simulink model "motor_simu"  (Simulink 7.7)
settings: Solver=ode45  StartTime=0.0  StopTime=100
values from neighbouring files (symbols this model uses):
  b = Cubesatmotorb    [main.m]
  J = Cubesatmotorrotorinertia    [main.m]
  Jc = structureinertiaJzz    [main.m]
  Jri = ((Cubesatmotorrotorinertia) + (flywheelinertiaJzz))    [main.m]
  Ke = CubesatmotorSconst    [main.m]
  Kt = CubesatmotorTconst    [main.m]
  L = CubesatmotorLrup    [main.m]
  R = CubesatmotorRrup    [main.m]
libraries: simulink x2
settings Model: Creator=Felipe  LastModifiedBy=user

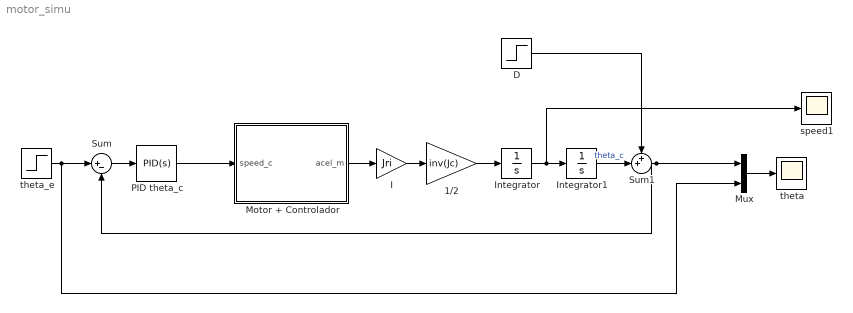
== system motor_simu ==
  1/2 : Gain  Gain=inv(Jc)
  D : Step  Time=150  After=(pi/4)/10  SampleTime=0
  I : Gain  Gain=Jri
  Integrator : Integrator
  Integrator1 : Integrator
  Motor + Controlador : Subsystem
  Mux : Mux  Inputs=2
  PID theta_c : simulink/Continuous/PID Controller  SystemSampleTime=-1  Controller=PID  TimeDomain=Continuous-time  SampleTime=1  IntegratorMethod=Forward Euler  FilterMethod=Forward Euler  Form=Parallel  P=4.2713440821133  I=0.2  D=-0.0891061021532855  N=47.9354834168987  InitialConditionSource=internal  InitialConditionForIntegrator=0  InitialConditionForFilter=0  ExternalReset=none  LimitOutput=off  UpperSaturationLimit=inf  LowerSaturationLimit=-inf  LinearizeAsGain=off  AntiWindupMode=none  Kb=1  TrackingMode=off  Kt=1  PParamMin=[]  PParamMax=[]  IParamMin=[]  IParamMax=[]  DParamMin=[]  DParamMax=[]  NParamMin=[]  NParamMax=[]  KbParamMin=[]  KbParamMax=[]  KtParamMin=[]  KtParamMax=[]  POutMin=[]  POutMax=[]  IOutMin=[]  IOutMax=[]  DOutMin=[]  DOutMax=[]  NOutMin=[]  NOutMax=[]  KbOutMin=[]  KbOutMax=[]  KtOutMin=[]  KtOutMax=[]  IntegratorOutMin=[]  IntegratorOutMax=[]  FilterOutMin=[]  FilterOutMax=[]  SumOutMin=[]  SumOutMax=[]  SumI1OutMin=[]  SumI1OutMax=[]  SumI2OutMin=[]  SumI2OutMax=[]  SumI3OutMin=[]  SumI3OutMax=[]  SumDOutMin=[]  SumDOutMax=[]  SaturationOutMin=[]  SaturationOutMax=[]  IntegratorContinuousStateAttributes=''  IntegratorStateMustResolveToSignalObject=off  IntegratorRTWStateStorageClass=Auto  FilterContinuousStateAttributes=''  FilterStateMustResolveToSignalObject=off  FilterRTWStateStorageClass=Auto
  Sum : Sum  Inputs=|+-
  Sum1 : Sum  Inputs=++|
  speed1 : Scope
      settings: SaveName=ScopeData3
  theta : Scope
      settings: YMin=-0.05  YMax=0.8
  theta_e : Step  After=(pi/4)  SampleTime=0
  wires:
  Motor + Controlador/1(acel_m) -> I/1
  I/1 -> 1/2/1
  Integrator/1 -> Integrator1/1, speed1/1
  PID theta_c/1 -> Motor + Controlador/1(speed_c)
  theta_e/1 -> Sum/1, Mux/2
  Sum/1 -> PID theta_c/1
  Mux/1 -> theta/1
  1/2/1 -> Integrator/1
  Integrator1/1 -> Sum1/2  "theta_c"
  D/1 -> Sum1/1
  Sum1/1 -> Sum/2, Mux/1

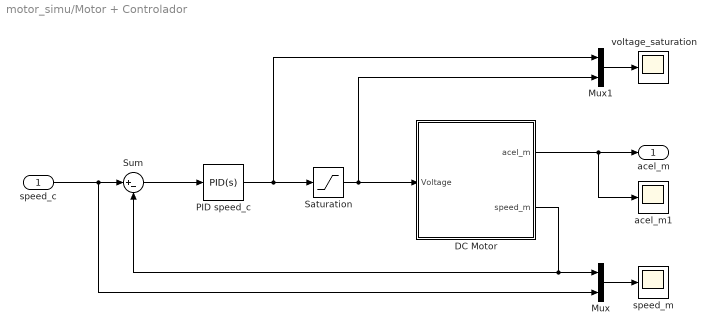
== system motor_simu/Motor + Controlador ==
  speed_c : Inport
  DC Motor : Subsystem
  Mux : Mux  Inputs=2
  Mux1 : Mux  Inputs=2
  PID speed_c : simulink/Continuous/PID Controller  SystemSampleTime=-1  Controller=PID  TimeDomain=Continuous-time  SampleTime=1  IntegratorMethod=Forward Euler  FilterMethod=Forward Euler  Form=Parallel  P=4.72772772635323  I=0.0083033953310603  D=-0.206120281132516  N=22.936742082715  InitialConditionSource=internal  InitialConditionForIntegrator=0  InitialConditionForFilter=0  ExternalReset=none  LimitOutput=off  UpperSaturationLimit=inf  LowerSaturationLimit=-inf  LinearizeAsGain=off  AntiWindupMode=none  Kb=1  TrackingMode=off  Kt=1  PParamMin=[]  PParamMax=[]  IParamMin=[]  IParamMax=[]  DParamMin=[]  DParamMax=[]  NParamMin=[]  NParamMax=[]  KbParamMin=[]  KbParamMax=[]  KtParamMin=[]  KtParamMax=[]  POutMin=[]  POutMax=[]  IOutMin=[]  IOutMax=[]  DOutMin=[]  DOutMax=[]  NOutMin=[]  NOutMax=[]  KbOutMin=[]  KbOutMax=[]  KtOutMin=[]  KtOutMax=[]  IntegratorOutMin=[]  IntegratorOutMax=[]  FilterOutMin=[]  FilterOutMax=[]  SumOutMin=[]  SumOutMax=[]  SumI1OutMin=[]  SumI1OutMax=[]  SumI2OutMin=[]  SumI2OutMax=[]  SumI3OutMin=[]  SumI3OutMax=[]  SumDOutMin=[]  SumDOutMax=[]  SaturationOutMin=[]  SaturationOutMax=[]  IntegratorContinuousStateAttributes=''  IntegratorStateMustResolveToSignalObject=off  IntegratorRTWStateStorageClass=Auto  FilterContinuousStateAttributes=''  FilterStateMustResolveToSignalObject=off  FilterRTWStateStorageClass=Auto
  Saturation : Saturate  UpperLimit=12  LowerLimit=-12
  Sum : Sum  Inputs=|+-
  acel_m1 : Scope
      settings: YMin=-0.095  YMax=0
  speed_m : Scope
      settings: SaveName=ScopeData2
  voltage_saturation : Scope
      settings: SaveName=ScopeData5
  acel_m : Outport
  wires:
  DC Motor/2(speed_m) -> Sum/2, Mux/1
  Saturation/1 -> DC Motor/1(Voltage), Mux1/2
  PID speed_c/1 -> Saturation/1, Mux1/1
  Sum/1 -> PID speed_c/1
  speed_c/1 -> Sum/1, Mux/2
  DC Motor/1(acel_m) -> acel_m/1, acel_m1/1
  Mux/1 -> speed_m/1
  Mux1/1 -> voltage_saturation/1

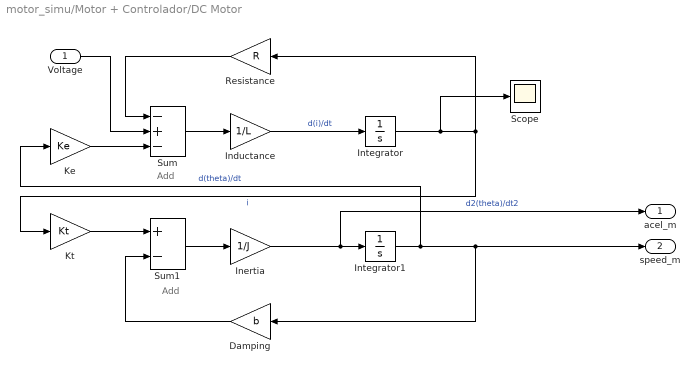
== system motor_simu/Motor + Controlador/DC Motor ==
  note: Add
  note: Add
  Voltage : Inport
  Damping : Gain  RequirementInfo={} %GIDa_a0bca8fb_deb2_4cd3_97cf_4f937a3969db  Gain=b
  Inductance : Gain  Gain=1/L
  Inertia : Gain  Gain=1/J
  Integrator : Integrator
  Integrator1 : Integrator
  Ke : Gain  Gain=Ke
  Kt : Gain  Gain=Kt
  Resistance : Gain  RequirementInfo={} %GIDa_06d63a89_88ab_48b6_b71f_14b802dc9c0a  Gain=R
  Scope : Scope
      settings: SaveName=ScopeData4
  Sum : Sum  Inputs=-+-
  Sum1 : Sum  Inputs=+-
  acel_m : Outport
  speed_m : Outport  Port=2
  wires:
  Resistance/1 -> Sum/1
  Voltage/1 -> Sum/2
  Ke/1 -> Sum/3
  Damping/1 -> Sum1/2
  Kt/1 -> Sum1/1
  Sum1/1 -> Inertia/1
  Sum/1 -> Inductance/1
  Inertia/1 -> Integrator1/1, acel_m/1  "d2(theta)/dt2"
  Integrator1/1 -> speed_m/1, Damping/1, Ke/1  "d(theta)/dt"
  Inductance/1 -> Integrator/1  "d(i)/dt"
  Integrator/1 -> Resistance/1, Kt/1, Scope/1  "i"
